simulink model "Modell"  (R2017b)
settings: Solver=VariableStepAuto  StartTime=0.0  StopTime=10.0  RelTol=1e-3
settings Model: Creator=arbno  LastModifiedBy=arbno

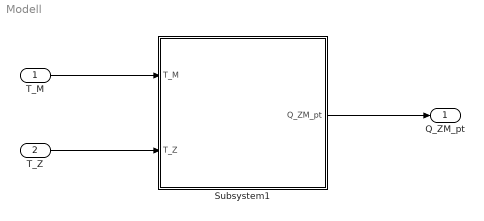
== system Modell ==
  T_M : Inport
  T_Z : Inport  Port=2
  Subsystem1 : Subsystem
  Q_ZM_pt : Outport
  wires:
  T_M/1 -> Subsystem1/1(T_M)
  T_Z/1 -> Subsystem1/2(T_Z)
  Subsystem1/1(Q_ZM_pt) -> Q_ZM_pt/1

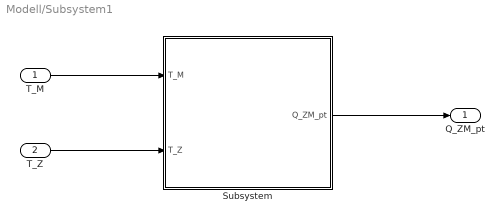
== system Modell/Subsystem1 ==
  T_M : Inport
  T_Z : Inport  Port=2
  Subsystem : Subsystem
  Q_ZM_pt : Outport
  wires:
  T_M/1 -> Subsystem/1(T_M)
  T_Z/1 -> Subsystem/2(T_Z)
  Subsystem/1(Q_ZM_pt) -> Q_ZM_pt/1

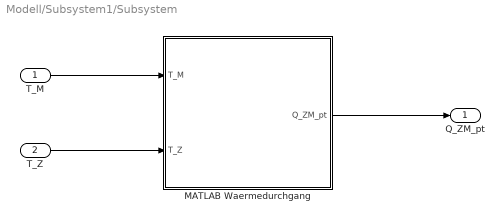
== system Modell/Subsystem1/Subsystem ==
  T_M : Inport
  T_Z : Inport  Port=2
  MATLAB Waermedurchgang : MATLAB Function  TreatAsAtomicUnit=on
  Q_ZM_pt : Outport
  wires:
  T_Z/1 -> MATLAB Waermedurchgang/2(T_Z)
  MATLAB Waermedurchgang/1(Q_ZM_pt) -> Q_ZM_pt/1
  T_M/1 -> MATLAB Waermedurchgang/1(T_M)

== matlab function Modell/Subsystem1/Subsystem/MATLAB Waermedurchgang ==
  data: Q_ZM_pt output; T_M input; T_Z input
function Q_ZM_pt =   Waermedurchgang(T_M, T_Z)
%#codegen
coder.extrinsic('IAPWS_IF97');
%Sattigungs dampfgehalt x_Dend

Q_ZM_pt = 0.5*(T_M - T_Z);

end
